simulink model "Test_lineargen_three_phase_pm_machine"  (Simulink 8.8)
settings: Solver=ode15s  StartTime=0.0  StopTime=5  RelTol=1e-3  EnableMultiTasking=on
libraries: powerlib x6, pm_machines_library x1
settings Model: SuppressorTable=22 serialization::archive 11 0 3 0 0 0 11 0  Creator=s0237326  LastModifiedBy=rcrozier
settings OptimizationCC: ExpressionDepthLimit=2147483647
settings DebuggingCC: SolverPrmCheckMsg=warning

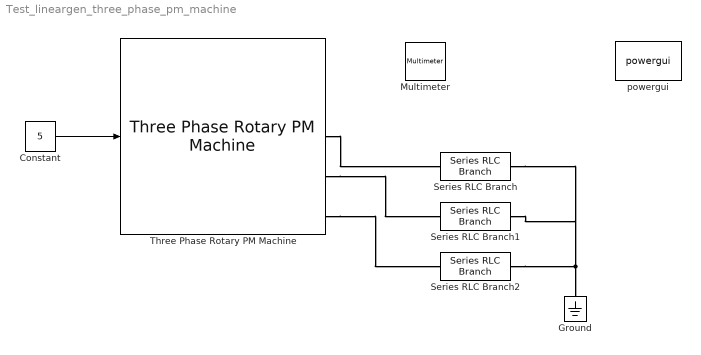
== system Test_lineargen_three_phase_pm_machine ==
  Constant : Constant  Value=5
  Ground : powerlib/Elements/Ground  LConnTagsString=a
  Multimeter : powerlib/Measurements/Multimeter  PhasorSimulation=off  OutputType=Complex  sel=[1 4 2 5 3 6]  L=6  Gain=[1 1 1 1 1 1]  yselected={'Ub: Series RLC Branch','Ib: Series RLC Branch','Ub: Series RLC Branch1','Ib: Series RLC Branch1','Ub: Series RLC Branch2','Ib: Series RLC Branch2'};  PSBOutputType=1  PSBequivalent=0  AxesSetting=[0,0.1,-100,100]  Display=1  SavedBlockNames=-11
  Series RLC Branch : powerlib/Elements/Series RLC Branch  LConnTagsString=__new0  RConnTagsString=__new0  BranchType=R  Resistance=100  Inductance=1e-3  SetiL0=off  InitialCurrent=0  Capacitance=1e-6  Setx0=off  InitialVoltage=0  Measurements=Branch voltage and current
  Series RLC Branch1 : powerlib/Elements/Series RLC Branch  LConnTagsString=__new0  RConnTagsString=__new0  BranchType=R  Resistance=100  Inductance=1e-3  SetiL0=off  InitialCurrent=0  Capacitance=1e-6  Setx0=off  InitialVoltage=0  Measurements=Branch voltage and current
  Series RLC Branch2 : powerlib/Elements/Series RLC Branch  LConnTagsString=__new0  RConnTagsString=__new0  BranchType=R  Resistance=100  Inductance=1e-3  SetiL0=off  InitialCurrent=0  Capacitance=1e-6  Setx0=off  InitialVoltage=0  Measurements=Branch voltage and current
  Three Phase Rotary PM Machine : pm_machines_library/Three Phase Rotary PM Machine  design_data_type_popup=From File  file_name_edit=test_lineargen_pm_machine_s_function.mat  design_workspace_edit=[]  simoptions_workspace_edit=[]
  powergui : powerlib/powergui  Priority=1  SimulationMode=Continuous  SolverType=Tustin/Backward Euler (TBE)  SampleTime=50e-6  frequency=60  SPID=off  DisableSnubberDevices=off  DisableRonSwitches=off  DisableVfSwitches=off  SwTol=0  DisplayEquations=off  Interpol=off  ExternalGateDelay=off  methode=off  Ts=10  FunctionMessages=off  echomessages=off  HookPort=off  EnableUseOfTLC=off  x0status=blocks  frequencyindice=0  Pbase=100e6  ErrMax=1e-4  Iterations=50  UnitsV=kV  UnitsW=MW  buscounter=0  RestoreLinks=warning  ResistiveCurrentMeasurement=off  Frange=[0:2:500]  Ylog=off  Xlog=on  ShowGrid=off  save=off  variable=ZData  structure=0  ZoomFFT=off  StartTime=0.0  cycles=1  DisplayStyle=1  fundamental=60  FreqAxis=off  MaxFrequency=1000  frequencyindicesteady=1  RmsSteady=1  display=off
  wires:
  Constant/1 -> Three Phase Rotary PM Machine/1
  connections:
  Series RLC Branch2/RConn1 -- Series RLC Branch/RConn1 -- Series RLC Branch1/RConn1 -- Ground/LConn1
  Three Phase Rotary PM Machine/RConn1 -- Series RLC Branch/LConn1
  Three Phase Rotary PM Machine/RConn2 -- Series RLC Branch1/LConn1
  Three Phase Rotary PM Machine/RConn3 -- Series RLC Branch2/LConn1
